simulink model "Model3"  (R2018b)
settings: Solver=VariableStepAuto  StartTime=0.0  StopTime=10.0  RelTol=1e-3
values from neighbouring files (symbols this model uses):
  a = 0.9    [dane.m]
  b = 1.07    [dane.m]
  c = 0.2773    [dane.m]
  d = 0.0026    [dane.m]
  g = 9.81    [ABS.m]    (also in dane.m)
  Jw = 0.01    [ABS.m]    (also in dane.m)
  mv = 1200    [ABS.m]    (also in dane.m)
  rw = 0.28    [ABS.m]    (also in dane.m = 0.3)
settings Model: Creator=Kasia  LastModifiedBy=Kasia

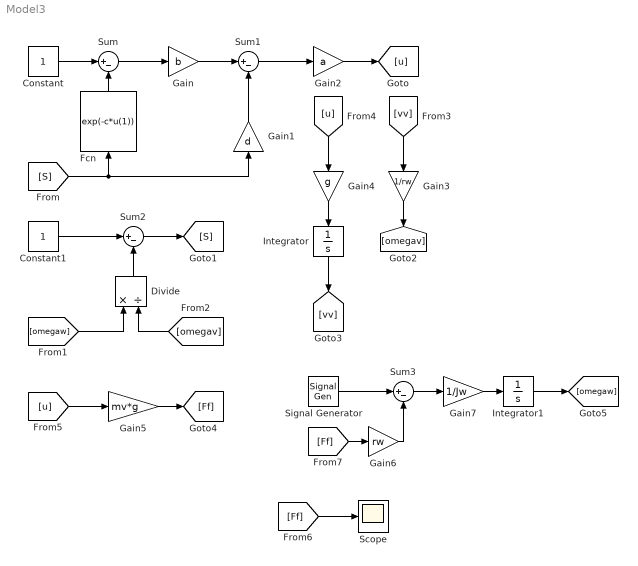
== system Model3 ==
  Constant : Constant
  Constant1 : Constant
  Divide : Product  Inputs=*/
  Fcn : Fcn  Expr=exp(-c*u(1))
  Gain : Gain  Gain=b
  Gain1 : Gain  Gain=d
  Gain2 : Gain  Gain=a
  Gain3 : Gain  Gain=1/rw
  Gain4 : Gain  Gain=g
  Gain5 : Gain  Gain=mv*g
  Gain6 : Gain  Gain=rw
  Gain7 : Gain  Gain=1/Jw
  Integrator : Integrator
  Integrator1 : Integrator  InitialCondition=1
  Scope : Scope
  Signal Generator : SignalGenerator  WaveForm=square  Amplitude=23  Units=rad/sec
  Sum{,1..3} (4 alike) : Sum  Inputs=|+-
  wires:
  Integrator1/1 -> [omegaw]
  Sum3/1 -> Gain7/1
  Gain1/1 -> Sum1/2
  [u] -> Gain5/1
  Gain7/1 -> Integrator1/1
  Gain5/1 -> [Ff]
  Sum1/1 -> Gain2/1
  Gain4/1 -> Integrator/1
  Integrator/1 -> [vv]
  [u] -> Gain4/1
  Sum2/1 -> [S]
  [omegav] -> Divide/2
  Constant1/1 -> Sum2/1
  [vv] -> Gain3/1
  Gain3/1 -> [omegav]
  Gain2/1 -> [u]
  Signal Generator/1 -> Sum3/1
  Divide/1 -> Sum2/2
  Fcn/1 -> Sum/2
  [S] -> Gain1/1, Fcn/1
  [omegaw] -> Divide/1
  [Ff] -> Gain6/1
  Gain6/1 -> Sum3/2
  Gain/1 -> Sum1/1
  Sum/1 -> Gain/1
  Constant/1 -> Sum/1
  [Ff] -> Scope/1
